simulink model "odeSolution"  (R2021a)
settings: Solver=VariableStepAuto  StartTime=0.0  StopTime=100  RelTol=1e-3
settings Model: Creator=Asus  LastModifiedBy=Asus

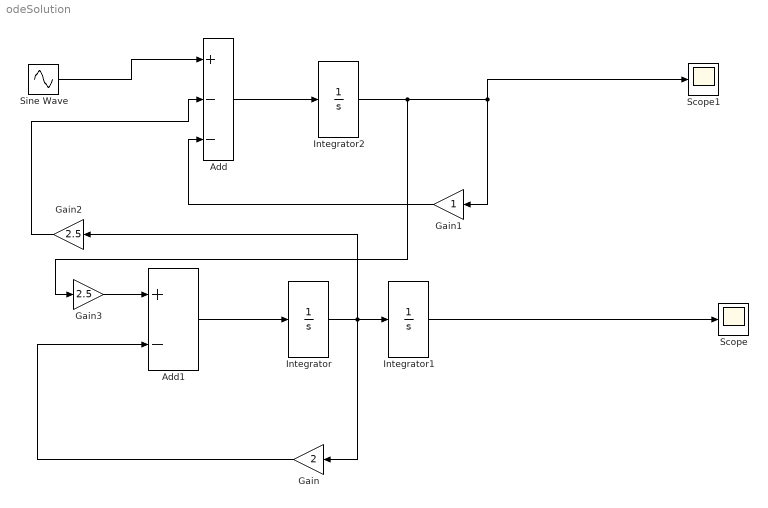
== system odeSolution ==
  Add : Sum  Inputs=+--
  Add1 : Sum  Inputs=+-
  Gain : Gain  Gain=2
  Gain1 : Gain
  Gain2 : Gain  Gain=2.5
  Gain3 : Gain  Gain=2.5
  Integrator : Integrator
  Integrator1 : Integrator
  Integrator2 : Integrator
  Scope : Scope
  Scope1 : Scope
  Sine Wave : Sin  Frequency=0.23  SampleTime=0
  wires:
  Sine Wave/1 -> Add/1
  Add1/1 -> Integrator/1
  Integrator/1 -> Gain2/1, Gain/1, Integrator1/1
  Gain/1 -> Add1/2
  Add/1 -> Integrator2/1
  Gain1/1 -> Add/3
  Integrator1/1 -> Scope/1
  Gain2/1 -> Add/2
  Gain3/1 -> Add1/1
  Integrator2/1 -> Gain3/1, Gain1/1, Scope1/1
